simulink model "two_tone_filter"  (R2025a)
settings: Solver=VariableStepAuto  StartTime=0.0  StopTime=10.0  RelTol=1e-3
PreLoadFcn:
  | PreprocIndata  = dataPreProc('data/sig_i.txt');
  | PreprocFirOutdata  = dataPreProc('data/fir_o.txt');
  | PreprocFftOutdata  = dataPreProc('data/fft_o.txt');
undefined symbols (not defined in the file or in its folder): FFT, FIR, i, L, None, vsva2197, xcvc1902
libraries: matrix_library x6, dspsrcs4 x3, aieDSP x2, aieUtilities x2, aieBasic x1, vmcUtilities x1
settings Model: Creator=ravidapu  LastModifiedBy=vkapadiy
settings DebuggingCC: UnconnectedInputMsg=warning  UnconnectedOutputMsg=warning  UnconnectedLineMsg=warning
settings ModelReferenceCC: EnableRefExpFcnMdlSchedulingChecks=on
settings RTWCC: GPUComputeCapability=3.5  DLArmComputeVersion=19.05

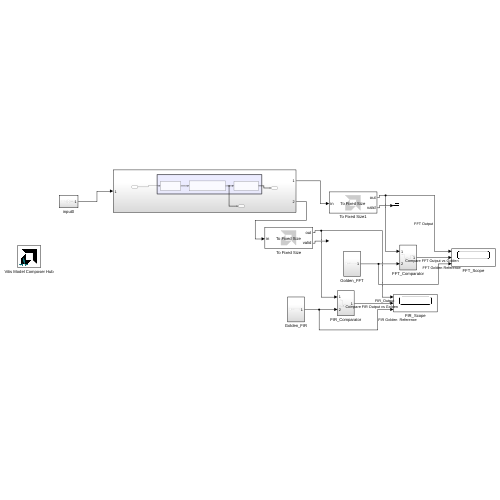
[thumbnail: Simulink's stored preview of the top-level diagram]
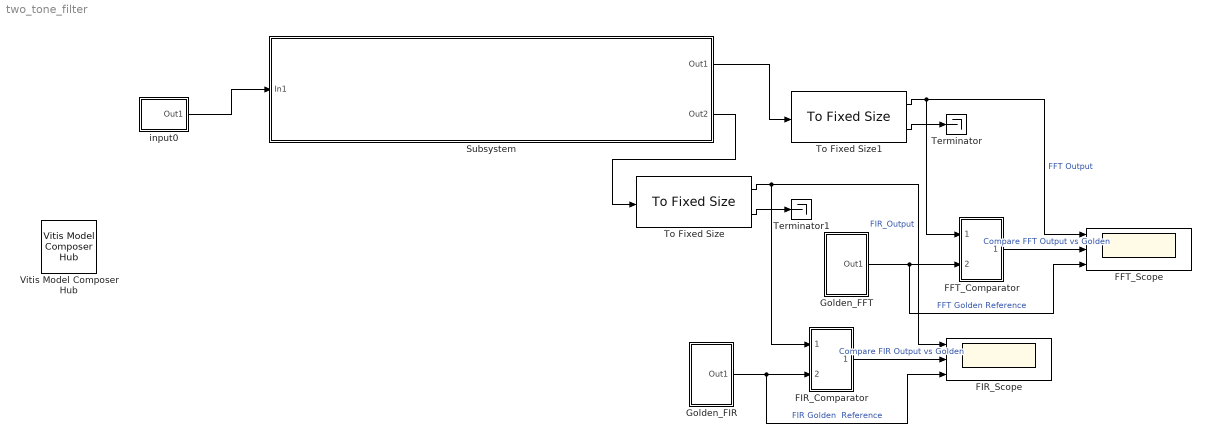
== system two_tone_filter ==
  FFT_Comparator : Subsystem
  FFT_Scope : Scope  NumInputPorts=3
      settings: ActiveDisplayYMinimum=-32768  ActiveDisplayYMaximum=32768
  FIR_Comparator : Subsystem
  FIR_Scope : Scope  NumInputPorts=3
      settings: ActiveDisplayYMinimum=-8558  ActiveDisplayYMaximum=11412
  Golden_FFT : Subsystem
  Golden_FIR : Subsystem
  Subsystem : Subsystem
  Terminator : Terminator
  Terminator1 : Terminator
  To Fixed Size : aieUtilities/To Fixed Size  Mode=Produce a valid output signal  OutputSize=2048  CopyMethod=Buffer samples to form output  HasStatusOutput=on
  To Fixed Size1 : aieUtilities/To Fixed Size  Mode=Produce a valid output signal  OutputSize=2048  CopyMethod=Buffer samples to form output  HasStatusOutput=on
  Vitis Model Composer Hub : vmcUtilities/Vitis Model Composer Hub  Tag=genX  CodeGeneration=off  SubsystemName=FIR-FFT  StartColumn=1  NumberOfColumns=1  TargetDirectory=./code  exportDesign=off  analyzeDesign=off  validateDesignOnHw=off  ExportType=AI Engines  IpVendor=xilinx.com  IpLibrary=hls  IpVersion=1.0  IpHWLanguage=Verilog  AieCompilerOptions={}  AieSimulatorOptions={}  AieGraphIterations=-1  CreateTestbench=on  TestbenchStackSize=10  RunRtlSim=off  RunCSim=off  RunAieSim=on  AieSimTimeout=50000  RunAieSimProfiling=off  LaunchVitisAnalyzer=on  PlotOutput=on  RunX86Sim=off  X86SimTimeout=10  GenHwImage=off  GenLibadfXo=off  GenHwValidationCode=off  PlatformType=Not Specified  HwSystemType=Baremetal  HwValidationTarget=hw  ProjDevice=xcvc1902-vsva2197-1LHP-i-L  ProjDevicePart=xcvc1902-vsva2197-1LHP-i-L  AIEType=AIE  SamplePeriod=-1  ClockFrequency=200  DataPathParallelism=1  xilinxfamily=versalaicore  part=xcvc1902  speed=-1LHP-i-L  package=vsva2197  directory=./netlist  testbench=off  incr_netlist=off  synthesis_tool=Vivado  clock_wrapper=Clock Enables  dbl_ovrd=According to Block Masks  dcm_input_clock_period=10  sysclk_period=10  simulink_period=1  eval_field=0  LogFileName=/group/techsup/cbalakr/github_cbalakr/my_projects/tsc_2023/ssr_lt1/vmc_demo/code/model_composer.log  NThreads=4
  input0 : Subsystem
  wires:
  Golden_FIR/1(Out1) -> FIR_Scope/3, FIR_Comparator/2(In2)  "FIR Golden  Reference"
  FFT_Comparator/1(Out1) -> FFT_Scope/2  "Compare FFT Output vs Golden"
  Golden_FFT/1(Out1) -> FFT_Scope/3, FFT_Comparator/2(In2)  "FFT Golden Reference"
  To Fixed Size1/1 -> FFT_Comparator/1(In1), FFT_Scope/1  "FFT Output"
  FIR_Comparator/1(Out1) -> FIR_Scope/2  "Compare FIR Output vs Golden"
  To Fixed Size/2 -> Terminator1/1
  To Fixed Size/1 -> FIR_Scope/1, FIR_Comparator/1(In1)  "FIR_Output"
  To Fixed Size1/2 -> Terminator/1
  input0/1(Out1) -> Subsystem/1(In1)
  Subsystem/1(Out1) -> To Fixed Size1/1
  Subsystem/2(Out2) -> To Fixed Size/1

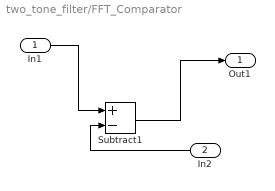
== system two_tone_filter/FFT_Comparator ==
  In1 : Inport
  In2 : Inport  Port=2
  Subtract1 : Sum  Inputs=+-  OutDataTypeStr=double
  Out1 : Outport
  wires:
  In1/1 -> Subtract1/1
  In2/1 -> Subtract1/2
  Subtract1/1 -> Out1/1

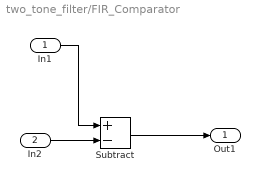
== system two_tone_filter/FIR_Comparator ==
  In1 : Inport
  In2 : Inport  Port=2
  Subtract : Sum  Inputs=+-
  Out1 : Outport
  wires:
  Subtract/1 -> Out1/1
  In2/1 -> Subtract/2
  In1/1 -> Subtract/1

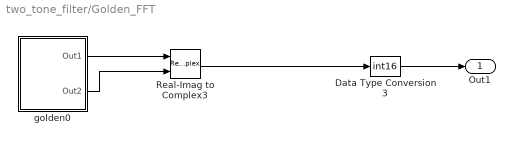
== system two_tone_filter/Golden_FFT ==
  Data Type Conversion3 : DataTypeConversion  OutDataTypeStr=int16  SaturateOnIntegerOverflow=off  RndMeth=Floor
  Real-Imag to Complex3 : RealImagToComplex
  golden0 : Subsystem
  Out1 : Outport
  wires:
  Real-Imag to Complex3/1 -> Data Type Conversion3/1
  golden0/2(Out2) -> Real-Imag to Complex3/2
  golden0/1(Out1) -> Real-Imag to Complex3/1
  Data Type Conversion3/1 -> Out1/1

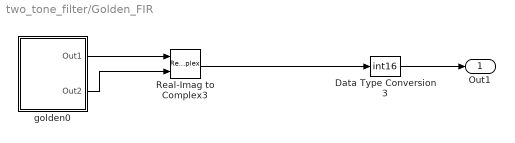
== system two_tone_filter/Golden_FIR ==
  Data Type Conversion3 : DataTypeConversion  OutDataTypeStr=int16  SaturateOnIntegerOverflow=off  RndMeth=Floor
  Real-Imag to Complex3 : RealImagToComplex
  golden0 : Subsystem
  Out1 : Outport
  wires:
  Real-Imag to Complex3/1 -> Data Type Conversion3/1
  golden0/2(Out2) -> Real-Imag to Complex3/2
  golden0/1(Out1) -> Real-Imag to Complex3/1
  Data Type Conversion3/1 -> Out1/1

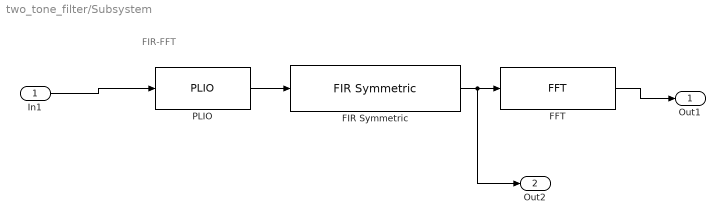
== system two_tone_filter/Subsystem ==
  note: FIR-FFT
  In1 : Inport
  FFT : aieDSP/FFT  AIE_VARIANT=1  data_type=cint16  data_out_type=cint16  twiddle_type=cint16  point_size=256  input_window_size=2048  shift_val=6  rnd_mode=Round to positive infinity  sat_mode=0-None  ssr=1  twiddle_mode=0  use_ssr_widget_kernels=off  casc_length=1  transform_fft_nifft=1  TP_API=0  TP_DYN_PT_SIZE=0  blockJsonConstraints=[]  blockJsonConstraintsInternal=[]  spec=vmc_fft.json  SerializedMaskParamNames=[]  SerializedMaskParamValues=[]  SerializedMaskParamVisibilities=[]  block_type=FFT  SerializedMaskParamDataypes=uint|typename|typename|typename|uint|uint|uint|uint|uint|uint|uint|uint|uint|uint|uint|uint  SerializedMaskParamEnumStrArr=0|0|0|0|0|0|0|Round to positive infinity,Round to negative infinity,Round symmetrical to infinity,Round symmetrical to zero,Round convergent to even,Round convergent to odd|0-None,1-Asymmetric,3-Symmetric|0|0|0|0|0|0|0  SerializedMaskParamEnumValArr=0|0|0|0|0|0|0|2,3,4,5,6,7|0,1,3|0|0|0|0|0|0|0  SerializedMaskParamVectorArr=0|0|0|0|0|0|0|0|0|0|0|0|0|0|0|0  SerializedMaskParamKeys=AIE_VARIANT|TT_DATA|TT_OUT_DATA|TT_TWIDDLE|TP_POINT_SIZE|TP_WINDOW_VSIZE|TP_SHIFT|TP_RND|TP_SAT|TP_PARALLEL_POWER|TP_TWIDDLE_MODE|TP_USE_WIDGETS|TP_CASC_LEN|TP_FFT_NIFFT|TP_API|TP_DYN_PT_SIZE
  FIR Symmetric : aieDSP/FIR Symmetric  data_type=cint16  coef_type=int16  use_coeff_reload=off  dual_ip=off  num_outputs=off  coeff=[25 19 -108 78 181 -376 19 734 -804 -562 2147 -1224 -3491 9535 20445]  fir_length=29  input_window_size=2048  shift_val=15  rnd_mode=Round to positive infinity  sat_mode=0-None  casc_length=1  AIE_VARIANT=1  TP_API=0  ssr=1  blockJsonConstraints=[]  blockJsonConstraintsInternal=[]  spec=vmc_fir_sr_sym.json  SerializedMaskParamNames=[]  SerializedMaskParamValues=[]  SerializedMaskParamVisibilities=[]  block_type=FIR Symmetric  SerializedMaskParamDataypes=typename|typename|uint|uint|uint|coef_type|uint|uint|uint|uint|uint|uint|uint|uint|uint  SerializedMaskParamEnumStrArr=0|0|0|0|0|0|0|0|0|Floor,Ceiling,Round to positive infinity,Round to negative infinity,Round symmetrical to infinity,Round symmetrical to zero,Round convergent to even,Round convergent to odd|0-None,1-Asymmetric,3-Symmetric|0|0|0|0  SerializedMaskParamEnumValArr=0|0|0|0|0|0|0|0|0|0,1,2,3,4,5,6,7|0,1,3|0|0|0|0  SerializedMaskParamVectorArr=0|0|0|0|0|1|0|0|0|0|0|0|0|0|0  SerializedMaskParamKeys=TT_DATA|TT_COEFF|TP_USE_COEFF_RELOAD|TP_DUAL_IP|TP_NUM_OUTPUTS|coeff|TP_FIR_LEN|TP_INPUT_WINDOW_VSIZE|TP_SHIFT|TP_RND|TP_SAT|TP_CASC_LEN|AIE_VARIANT|TP_API|TP_SSR
  PLIO : aieBasic/PLIO  PlioWidth=64  PlioFreqSpec=off  PlioFreq=250  ColLocation=0  channel=0  blockJsonConstraints=[]  deprecateConstraints=0
  Out1 : Outport
  Out2 : Outport  Port=2
  wires:
  PLIO/1 -> FIR Symmetric/1
  In1/1 -> PLIO/1
  FFT/1 -> Out1/1
  FIR Symmetric/1 -> Out2/1, FFT/1

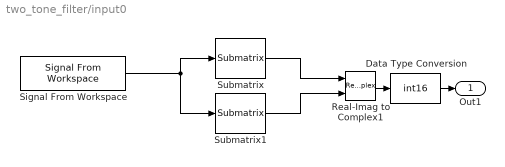
== system two_tone_filter/input0 ==
  Data Type Conversion : DataTypeConversion  OutDataTypeStr=int16  SaturateOnIntegerOverflow=off  RndMeth=Floor
  Real-Imag to Complex1 : RealImagToComplex
  Signal From Workspace : dspsrcs4/Signal From Workspace  X=PreprocIndata  Ts=1  nsamps=2048  OutputAfterFinalValue=Setting to zero  ignoreOrWarnInputAndFrameLengths=off  OutputFrames=off
  Submatrix : matrix_library/Submatrix  RowSpan=All rows  RowStartMode=First  RowStartIndex=1  RowEndMode=Last  RowEndIndex=1  ColSpan=One column  ColStartMode=First  ColStartIndex=1  ColEndMode=Last  ColEndIndex=1
  Submatrix1 : matrix_library/Submatrix  RowSpan=All rows  RowStartMode=First  RowStartIndex=1  RowEndMode=Last  RowEndIndex=1  ColSpan=One column  ColStartMode=Last  ColStartIndex=1  ColEndMode=Last  ColEndIndex=1
  Out1 : Outport
  wires:
  Signal From Workspace/1 -> Submatrix1/1, Submatrix/1
  Submatrix/1 -> Real-Imag to Complex1/1
  Submatrix1/1 -> Real-Imag to Complex1/2
  Real-Imag to Complex1/1 -> Data Type Conversion/1
  Data Type Conversion/1 -> Out1/1

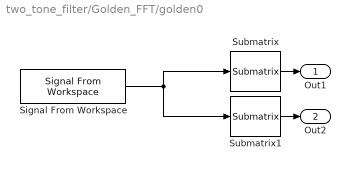
== system two_tone_filter/Golden_FFT/golden0 ==
  Signal From Workspace : dspsrcs4/Signal From Workspace  X=PreprocFftOutdata  Ts=1  nsamps=2048  OutputAfterFinalValue=Setting to zero  ignoreOrWarnInputAndFrameLengths=on  OutputFrames=off
  Submatrix : matrix_library/Submatrix  RowSpan=All rows  RowStartMode=First  RowStartIndex=1  RowEndMode=Last  RowEndIndex=1  ColSpan=One column  ColStartMode=First  ColStartIndex=1  ColEndMode=Last  ColEndIndex=1
  Submatrix1 : matrix_library/Submatrix  RowSpan=All rows  RowStartMode=First  RowStartIndex=1  RowEndMode=Last  RowEndIndex=1  ColSpan=One column  ColStartMode=Last  ColStartIndex=1  ColEndMode=Last  ColEndIndex=1
  Out1 : Outport  VectorParamsAs1DForOutWhenUnconnected=off
  Out2 : Outport  Port=2  VectorParamsAs1DForOutWhenUnconnected=off
  wires:
  Submatrix/1 -> Out1/1
  Signal From Workspace/1 -> Submatrix/1, Submatrix1/1
  Submatrix1/1 -> Out2/1

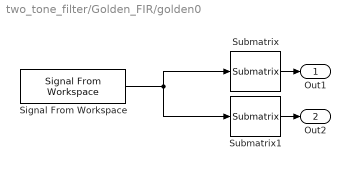
== system two_tone_filter/Golden_FIR/golden0 ==
  Signal From Workspace : dspsrcs4/Signal From Workspace  X=PreprocFirOutdata  Ts=1  nsamps=2048  OutputAfterFinalValue=Setting to zero  ignoreOrWarnInputAndFrameLengths=on  OutputFrames=off
  Submatrix : matrix_library/Submatrix  RowSpan=All rows  RowStartMode=First  RowStartIndex=1  RowEndMode=Last  RowEndIndex=1  ColSpan=One column  ColStartMode=First  ColStartIndex=1  ColEndMode=Last  ColEndIndex=1
  Submatrix1 : matrix_library/Submatrix  RowSpan=All rows  RowStartMode=First  RowStartIndex=1  RowEndMode=Last  RowEndIndex=1  ColSpan=One column  ColStartMode=Last  ColStartIndex=1  ColEndMode=Last  ColEndIndex=1
  Out1 : Outport  VectorParamsAs1DForOutWhenUnconnected=off
  Out2 : Outport  Port=2  VectorParamsAs1DForOutWhenUnconnected=off
  wires:
  Submatrix/1 -> Out1/1
  Signal From Workspace/1 -> Submatrix/1, Submatrix1/1
  Submatrix1/1 -> Out2/1
